simulink model "CP_SFC_Lin_b_n9945008"  (R2018b)
settings: Solver=ode4  StartTime=0.0  StopTime=5  FixedStep=0.02  RelTol=1e-3
values from neighbouring files (symbols this model uses):
  Ab = [ 0 ,        0           , 1 , 0 ... (first row only)    [CP_SFC_Lin_b_MainFile_n9945008.m]
  Bb = [0;0;1/Mc;1/(l*Mc)]    [CP_SFC_Lin_b_MainFile_n9945008.m]
  Cb = eye(4)    [CP_SFC_Lin_b_MainFile_n9945008.m]
  Db = zeros(4,1)    [CP_SFC_Lin_b_MainFile_n9945008.m]
  Kb = place(Ab,Bb, [-3,-4,-5,-6])    [CP_SFC_Lin_b_MainFile_n9945008.m]
  setPoint = pi    (= 3.14159265359)    [CP_SFC_Lin_b_MainFile_n9945008.m]
  x0 = [0.2 20*pi/180 0 0]'    [CP_SFC_Lin_a_MainFile_n9945008.m]    (also in CP_SFC_Lin_b_MainFile_n9945008.m = [0.4 200*pi/180 0 0]')
settings Model: Creator=Cody  LastModifiedBy=Cody

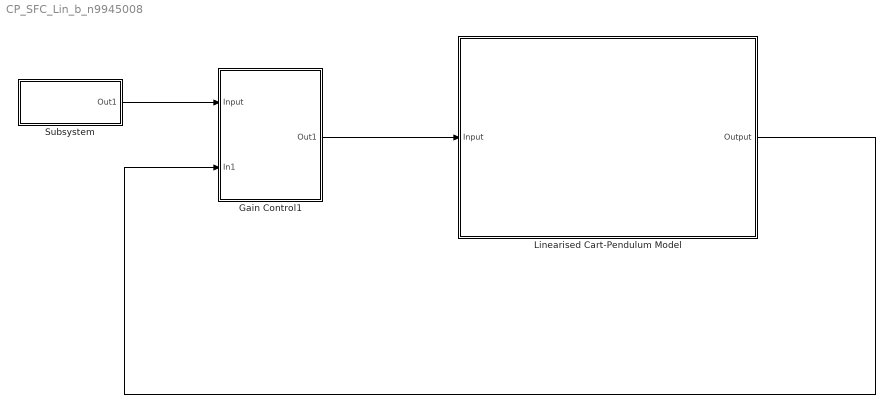
== system CP_SFC_Lin_b_n9945008 ==
  Gain Control1 : Subsystem
  "Linearised Cart-Pendulum Model " : Subsystem
  Subsystem : Subsystem
  wires:
  Gain Control1/1(Out1) -> "Linearised Cart-Pendulum Model "/1(Input)
  "Linearised Cart-Pendulum Model "/1(Output) -> Gain Control1/2(In1)
  Subsystem/1(Out1) -> Gain Control1/1(Input)

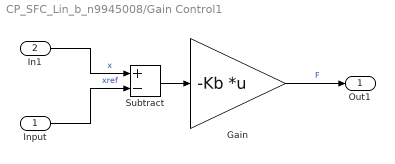
== system CP_SFC_Lin_b_n9945008/Gain Control1 ==
  Input : Inport
  In1 : Inport  Port=2
  Gain : Gain  Gain=-Kb  Multiplication=Matrix(K*u)
  Subtract : Sum  Inputs=+-
  Out1 : Outport
  wires:
  Gain/1 -> Out1/1  "F"
  In1/1 -> Subtract/1  "x"
  Input/1 -> Subtract/2  "xref"
  Subtract/1 -> Gain/1

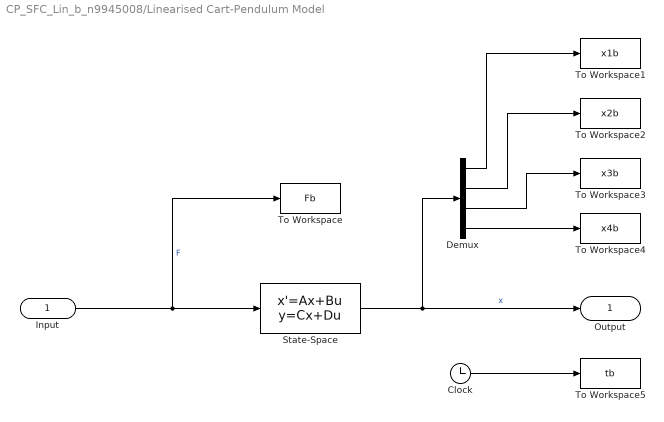
== system CP_SFC_Lin_b_n9945008/Linearised Cart-Pendulum Model  ==
  Input : Inport
  Clock : Clock
  Demux : Demux
  State-Space : StateSpace  A=Ab  B=Bb  C=Cb  D=Db  InitialCondition=x0
  To Workspace : ToWorkspace  VariableName=Fb  SampleTime=-1
      settings: Save2DSignal=2-D array (concatenate along first dimension)
  To Workspace1 : ToWorkspace  VariableName=x1b  SampleTime=-1
      settings: Save2DSignal=2-D array (concatenate along first dimension)
  To Workspace2 : ToWorkspace  VariableName=x2b  SampleTime=-1
      settings: Save2DSignal=2-D array (concatenate along first dimension)
  To Workspace3 : ToWorkspace  VariableName=x3b  SampleTime=-1
      settings: Save2DSignal=2-D array (concatenate along first dimension)
  To Workspace4 : ToWorkspace  VariableName=x4b  SampleTime=-1
      settings: Save2DSignal=2-D array (concatenate along first dimension)
  To Workspace5 : ToWorkspace  VariableName=tb  SampleTime=-1
      settings: Save2DSignal=2-D array (concatenate along first dimension)
  Output : Outport
  wires:
  Clock/1 -> To Workspace5/1
  Demux/1 -> To Workspace1/1
  State-Space/1 -> Demux/1, Output/1  "x"
  Demux/4 -> To Workspace4/1
  Input/1 -> To Workspace/1, State-Space/1  "F"
  Demux/2 -> To Workspace2/1
  Demux/3 -> To Workspace3/1

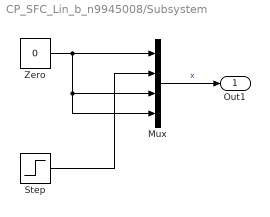
== system CP_SFC_Lin_b_n9945008/Subsystem ==
  Mux : Mux
  Step : Step  Time=0  After=setPoint  SampleTime=0
  Zero : Constant  Value=0  OutDataTypeStr=Inherit: Inherit via back propagation
  Out1 : Outport
  wires:
  Mux/1 -> Out1/1  "x"
  Zero/1 -> Mux/4, Mux/3, Mux/1
  Step/1 -> Mux/2
